simulink model "dvoukompar"  (Simulink 8.0)
settings: Solver=ode45  StartTime=0.0  StopTime=100  RelTol=1e-3
settings Model: Creator=polacmi1  LastModifiedBy=Jarda
settings DataIOCC: SignalLoggingSaveFormat=ModelDataLogs
settings DebuggingCC: FcnCallInpInsideContextMsg=EnableAllAsWarning

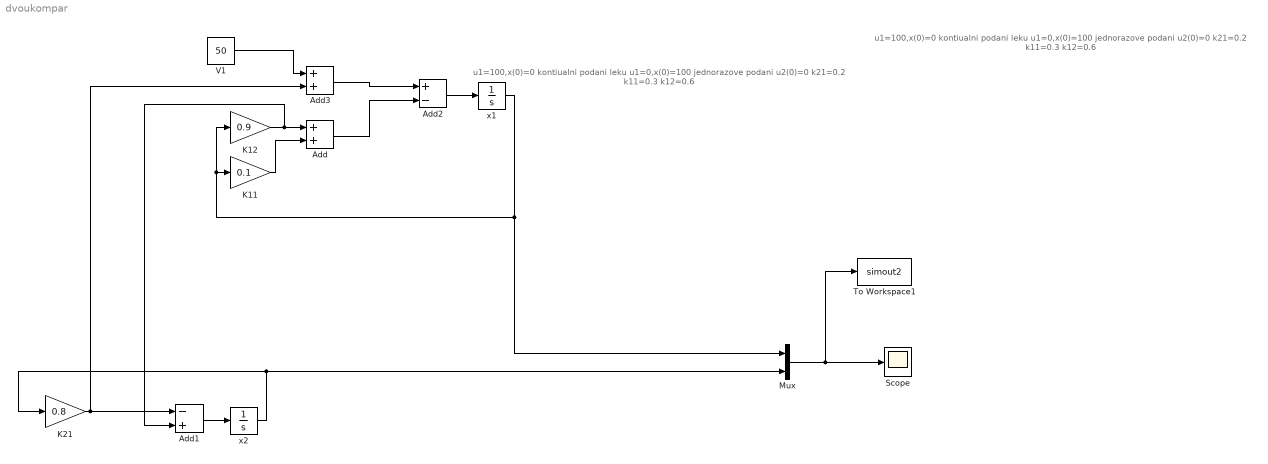
== system dvoukompar ==
  note: u1=100,x(0)=0 kontiualni podani leku
      | u1=0,x(0)=100 jednorazove podani
      | u2(0)=0
      | k21=0.2
      | k11=0.3
      | k12=0.6
  note: u1=100,x(0)=0 kontiualni podani leku
      | u1=0,x(0)=100 jednorazove podani
      | u2(0)=0
      | k21=0.2
      | k11=0.3
      | k12=0.6
  Add : Sum
  Add1 : Sum  Inputs=-+
  Add2 : Sum  Inputs=+-
  Add3 : Sum
  K11 : Gain  Gain=0.1
  K12 : Gain  Gain=0.9
  K21 : Gain  Gain=0.8
  Mux : Mux  Inputs=2
  Scope : Scope
      settings: DataFormat=Structure
  To Workspace1 : ToWorkspace  VariableName=simout2  SampleTime=-1  SaveFormat=Timeseries
  V1 : Constant  Value=50
  x1 : Integrator
  x2 : Integrator
  wires:
  K11/1 -> Add/2
  x2/1 -> K21/1, Mux/2
  Add1/1 -> x2/1
  Add2/1 -> x1/1
  Add/1 -> Add2/2
  K12/1 -> Add/1, Add1/2
  V1/1 -> Add3/1
  K21/1 -> Add3/2, Add1/1
  Add3/1 -> Add2/1
  Mux/1 -> To Workspace1/1, Scope/1
  x1/1 -> K11/1, K12/1, Mux/1
